simulink model "c00010M_harness"  (R2018a)
settings: Solver=FixedStepAuto  StartTime=0.0  StopTime=300  FixedStep=0.1  RelTol=1e-3
undefined symbols (not defined in the file): A1, hmax, PriorityTank, R1, R2, sigbuilder_block, TempThreshold
(part 5 of 40)

== system c00010M_harness/M143 ==
  note: VALUES
      | ---------------------------------
      | ControlType = 1 | 2 | 3
      | FillTank = 0 | 1
      | EmptyTank = 0 | 1
      | ManualReference between 0 and 1
      | Tempreature between 0 and 100
      | EmergencyButton = 0 | 1
      | LiquidLevel between 0 and 1 (hmax)
  note: Inputs For Tank2
  note: NAMES
      | --------------------------------------------
      | CT1 = ControlType Tank 1
      | F1 = Fill Tank 1
      | E1 = Empty Tank 1
      | MR1 = Manual Reference Tank1
      | T1 = Temperature Tank 1
      | EB1 = Emergency Button Tank 1
      | LL1 = Liquid Level 1
  note: Inputs For Tank3
  note: Inputs For Tank1
  CT2 : Inport
  F2 : Inport  Port=2
  E2 : Inport  Port=3
  T2 : Inport  Port=4
  EB2 : Inport  Port=5
  CT3 : Inport  Port=6
  F3 : Inport  Port=7
  E3 : Inport  Port=8
  MR3 : Inport  Port=9
  T3 : Inport  Port=10
  EB3 : Inport  Port=11
  Tank2 : Subsystem
  Tank3 : Subsystem
  LL2 : Outport
  LL3 : Outport  Port=2
  wires:
  Tank2/1(LL2) -> LL2/1, Tank3/7(LL2)
  Tank3/1(LL3) -> LL3/1, Tank2/6(LL3)
  EB2/1 -> Tank2/5(EB2)
  MR3/1 -> Tank3/4(MR3)
  CT2/1 -> Tank2/1(CT2)
  F2/1 -> Tank2/2(F2)
  E3/1 -> Tank3/3(E3)
  E2/1 -> Tank2/3(E2)
  T2/1 -> Tank2/4(T2)
  CT3/1 -> Tank3/1(CT3)
  F3/1 -> Tank3/2(F3)
  EB3/1 -> Tank3/6(EB3)
  T3/1 -> Tank3/5(T3)

== system c00010M_harness/M144 ==
  note: VALUES
      | ---------------------------------
      | ControlType = 1 | 2 | 3
      | FillTank = 0 | 1
      | EmptyTank = 0 | 1
      | ManualReference between 0 and 1
      | Tempreature between 0 and 100
      | EmergencyButton = 0 | 1
      | LiquidLevel between 0 and 1 (hmax)
  note: Inputs For Tank2
  note: NAMES
      | --------------------------------------------
      | CT1 = ControlType Tank 1
      | F1 = Fill Tank 1
      | E1 = Empty Tank 1
      | MR1 = Manual Reference Tank1
      | T1 = Temperature Tank 1
      | EB1 = Emergency Button Tank 1
      | LL1 = Liquid Level 1
  note: Inputs For Tank3
  note: Inputs For Tank1
  CT2 : Inport
  F2 : Inport  Port=2
  E2 : Inport  Port=3
  T2 : Inport  Port=4
  EB2 : Inport  Port=5
  CT3 : Inport  Port=6
  F3 : Inport  Port=7
  E3 : Inport  Port=8
  MR3 : Inport  Port=9
  T3 : Inport  Port=10
  EB3 : Inport  Port=11
  Tank2 : Subsystem
  Tank3 : Subsystem
  LL2 : Outport
  LL3 : Outport  Port=2
  wires:
  Tank2/1(LL2) -> LL2/1, Tank3/7(LL2)
  Tank3/1(LL3) -> LL3/1, Tank2/6(LL3)
  EB2/1 -> Tank2/5(EB2)
  MR3/1 -> Tank3/4(MR3)
  CT2/1 -> Tank2/1(CT2)
  F2/1 -> Tank2/2(F2)
  E3/1 -> Tank3/3(E3)
  E2/1 -> Tank2/3(E2)
  T2/1 -> Tank2/4(T2)
  CT3/1 -> Tank3/1(CT3)
  F3/1 -> Tank3/2(F3)
  EB3/1 -> Tank3/6(EB3)
  T3/1 -> Tank3/5(T3)

== system c00010M_harness/M145 ==
  note: VALUES
      | ---------------------------------
      | ControlType = 1 | 2 | 3
      | FillTank = 0 | 1
      | EmptyTank = 0 | 1
      | ManualReference between 0 and 1
      | Tempreature between 0 and 100
      | EmergencyButton = 0 | 1
      | LiquidLevel between 0 and 1 (hmax)
  note: Inputs For Tank2
  note: NAMES
      | --------------------------------------------
      | CT1 = ControlType Tank 1
      | F1 = Fill Tank 1
      | E1 = Empty Tank 1
      | MR1 = Manual Reference Tank1
      | T1 = Temperature Tank 1
      | EB1 = Emergency Button Tank 1
      | LL1 = Liquid Level 1
  note: Inputs For Tank3
  note: Inputs For Tank1
  CT2 : Inport
  F2 : Inport  Port=2
  E2 : Inport  Port=3
  T2 : Inport  Port=4
  EB2 : Inport  Port=5
  CT3 : Inport  Port=6
  F3 : Inport  Port=7
  E3 : Inport  Port=8
  MR3 : Inport  Port=9
  T3 : Inport  Port=10
  EB3 : Inport  Port=11
  Tank2 : Subsystem
  Tank3 : Subsystem
  LL2 : Outport
  LL3 : Outport  Port=2
  wires:
  Tank2/1(LL2) -> LL2/1, Tank3/7(LL2)
  Tank3/1(LL3) -> LL3/1, Tank2/6(LL3)
  EB2/1 -> Tank2/5(EB2)
  MR3/1 -> Tank3/4(MR3)
  CT2/1 -> Tank2/1(CT2)
  F2/1 -> Tank2/2(F2)
  E3/1 -> Tank3/3(E3)
  E2/1 -> Tank2/3(E2)
  T2/1 -> Tank2/4(T2)
  CT3/1 -> Tank3/1(CT3)
  F3/1 -> Tank3/2(F3)
  EB3/1 -> Tank3/6(EB3)
  T3/1 -> Tank3/5(T3)

== system c00010M_harness/M146 ==
  note: VALUES
      | ---------------------------------
      | ControlType = 1 | 2 | 3
      | FillTank = 0 | 1
      | EmptyTank = 0 | 1
      | ManualReference between 0 and 1
      | Tempreature between 0 and 100
      | EmergencyButton = 0 | 1
      | LiquidLevel between 0 and 1 (hmax)
  note: Inputs For Tank2
  note: NAMES
      | --------------------------------------------
      | CT1 = ControlType Tank 1
      | F1 = Fill Tank 1
      | E1 = Empty Tank 1
      | MR1 = Manual Reference Tank1
      | T1 = Temperature Tank 1
      | EB1 = Emergency Button Tank 1
      | LL1 = Liquid Level 1
  note: Inputs For Tank3
  note: Inputs For Tank1
  CT2 : Inport
  F2 : Inport  Port=2
  E2 : Inport  Port=3
  T2 : Inport  Port=4
  EB2 : Inport  Port=5
  CT3 : Inport  Port=6
  F3 : Inport  Port=7
  E3 : Inport  Port=8
  MR3 : Inport  Port=9
  T3 : Inport  Port=10
  EB3 : Inport  Port=11
  Tank2 : Subsystem
  Tank3 : Subsystem
  LL2 : Outport
  LL3 : Outport  Port=2
  wires:
  Tank2/1(LL2) -> LL2/1, Tank3/7(LL2)
  Tank3/1(LL3) -> LL3/1, Tank2/6(LL3)
  EB2/1 -> Tank2/5(EB2)
  MR3/1 -> Tank3/4(MR3)
  CT2/1 -> Tank2/1(CT2)
  F2/1 -> Tank2/2(F2)
  E3/1 -> Tank3/3(E3)
  E2/1 -> Tank2/3(E2)
  T2/1 -> Tank2/4(T2)
  CT3/1 -> Tank3/1(CT3)
  F3/1 -> Tank3/2(F3)
  EB3/1 -> Tank3/6(EB3)
  T3/1 -> Tank3/5(T3)

== system c00010M_harness/M147 ==
  note: VALUES
      | ---------------------------------
      | ControlType = 1 | 2 | 3
      | FillTank = 0 | 1
      | EmptyTank = 0 | 1
      | ManualReference between 0 and 1
      | Tempreature between 0 and 100
      | EmergencyButton = 0 | 1
      | LiquidLevel between 0 and 1 (hmax)
  note: Inputs For Tank2
  note: NAMES
      | --------------------------------------------
      | CT1 = ControlType Tank 1
      | F1 = Fill Tank 1
      | E1 = Empty Tank 1
      | MR1 = Manual Reference Tank1
      | T1 = Temperature Tank 1
      | EB1 = Emergency Button Tank 1
      | LL1 = Liquid Level 1
  note: Inputs For Tank3
  note: Inputs For Tank1
  CT2 : Inport
  F2 : Inport  Port=2
  E2 : Inport  Port=3
  T2 : Inport  Port=4
  EB2 : Inport  Port=5
  CT3 : Inport  Port=6
  F3 : Inport  Port=7
  E3 : Inport  Port=8
  MR3 : Inport  Port=9
  T3 : Inport  Port=10
  EB3 : Inport  Port=11
  Tank2 : Subsystem
  Tank3 : Subsystem
  LL2 : Outport
  LL3 : Outport  Port=2
  wires:
  Tank2/1(LL2) -> LL2/1, Tank3/7(LL2)
  Tank3/1(LL3) -> LL3/1, Tank2/6(LL3)
  EB2/1 -> Tank2/5(EB2)
  MR3/1 -> Tank3/4(MR3)
  CT2/1 -> Tank2/1(CT2)
  F2/1 -> Tank2/2(F2)
  E3/1 -> Tank3/3(E3)
  E2/1 -> Tank2/3(E2)
  T2/1 -> Tank2/4(T2)
  CT3/1 -> Tank3/1(CT3)
  F3/1 -> Tank3/2(F3)
  EB3/1 -> Tank3/6(EB3)
  T3/1 -> Tank3/5(T3)

== system c00010M_harness/M148 ==
  note: VALUES
      | ---------------------------------
      | ControlType = 1 | 2 | 3
      | FillTank = 0 | 1
      | EmptyTank = 0 | 1
      | ManualReference between 0 and 1
      | Tempreature between 0 and 100
      | EmergencyButton = 0 | 1
      | LiquidLevel between 0 and 1 (hmax)
  note: Inputs For Tank2
  note: NAMES
      | --------------------------------------------
      | CT1 = ControlType Tank 1
      | F1 = Fill Tank 1
      | E1 = Empty Tank 1
      | MR1 = Manual Reference Tank1
      | T1 = Temperature Tank 1
      | EB1 = Emergency Button Tank 1
      | LL1 = Liquid Level 1
  note: Inputs For Tank3
  note: Inputs For Tank1
  CT2 : Inport
  F2 : Inport  Port=2
  E2 : Inport  Port=3
  T2 : Inport  Port=4
  EB2 : Inport  Port=5
  CT3 : Inport  Port=6
  F3 : Inport  Port=7
  E3 : Inport  Port=8
  MR3 : Inport  Port=9
  T3 : Inport  Port=10
  EB3 : Inport  Port=11
  Tank2 : Subsystem
  Tank3 : Subsystem
  LL2 : Outport
  LL3 : Outport  Port=2
  wires:
  Tank2/1(LL2) -> LL2/1, Tank3/7(LL2)
  Tank3/1(LL3) -> LL3/1, Tank2/6(LL3)
  EB2/1 -> Tank2/5(EB2)
  MR3/1 -> Tank3/4(MR3)
  CT2/1 -> Tank2/1(CT2)
  F2/1 -> Tank2/2(F2)
  E3/1 -> Tank3/3(E3)
  E2/1 -> Tank2/3(E2)
  T2/1 -> Tank2/4(T2)
  CT3/1 -> Tank3/1(CT3)
  F3/1 -> Tank3/2(F3)
  EB3/1 -> Tank3/6(EB3)
  T3/1 -> Tank3/5(T3)

== system c00010M_harness/M149 ==
  note: VALUES
      | ---------------------------------
      | ControlType = 1 | 2 | 3
      | FillTank = 0 | 1
      | EmptyTank = 0 | 1
      | ManualReference between 0 and 1
      | Tempreature between 0 and 100
      | EmergencyButton = 0 | 1
      | LiquidLevel between 0 and 1 (hmax)
  note: Inputs For Tank2
  note: NAMES
      | --------------------------------------------
      | CT1 = ControlType Tank 1
      | F1 = Fill Tank 1
      | E1 = Empty Tank 1
      | MR1 = Manual Reference Tank1
      | T1 = Temperature Tank 1
      | EB1 = Emergency Button Tank 1
      | LL1 = Liquid Level 1
  note: Inputs For Tank3
  note: Inputs For Tank1
  CT2 : Inport
  F2 : Inport  Port=2
  E2 : Inport  Port=3
  T2 : Inport  Port=4
  EB2 : Inport  Port=5
  CT3 : Inport  Port=6
  F3 : Inport  Port=7
  E3 : Inport  Port=8
  MR3 : Inport  Port=9
  T3 : Inport  Port=10
  EB3 : Inport  Port=11
  Tank2 : Subsystem
  Tank3 : Subsystem
  LL2 : Outport
  LL3 : Outport  Port=2
  wires:
  Tank2/1(LL2) -> LL2/1, Tank3/7(LL2)
  Tank3/1(LL3) -> LL3/1, Tank2/6(LL3)
  EB2/1 -> Tank2/5(EB2)
  MR3/1 -> Tank3/4(MR3)
  CT2/1 -> Tank2/1(CT2)
  F2/1 -> Tank2/2(F2)
  E3/1 -> Tank3/3(E3)
  E2/1 -> Tank2/3(E2)
  T2/1 -> Tank2/4(T2)
  CT3/1 -> Tank3/1(CT3)
  F3/1 -> Tank3/2(F3)
  EB3/1 -> Tank3/6(EB3)
  T3/1 -> Tank3/5(T3)

== system c00010M_harness/M150 ==
  note: VALUES
      | ---------------------------------
      | ControlType = 1 | 2 | 3
      | FillTank = 0 | 1
      | EmptyTank = 0 | 1
      | ManualReference between 0 and 1
      | Tempreature between 0 and 100
      | EmergencyButton = 0 | 1
      | LiquidLevel between 0 and 1 (hmax)
  note: Inputs For Tank2
  note: NAMES
      | --------------------------------------------
      | CT1 = ControlType Tank 1
      | F1 = Fill Tank 1
      | E1 = Empty Tank 1
      | MR1 = Manual Reference Tank1
      | T1 = Temperature Tank 1
      | EB1 = Emergency Button Tank 1
      | LL1 = Liquid Level 1
  note: Inputs For Tank3
  note: Inputs For Tank1
  CT2 : Inport
  F2 : Inport  Port=2
  E2 : Inport  Port=3
  T2 : Inport  Port=4
  EB2 : Inport  Port=5
  CT3 : Inport  Port=6
  F3 : Inport  Port=7
  E3 : Inport  Port=8
  MR3 : Inport  Port=9
  T3 : Inport  Port=10
  EB3 : Inport  Port=11
  Tank2 : Subsystem
  Tank3 : Subsystem
  LL2 : Outport
  LL3 : Outport  Port=2
  wires:
  Tank2/1(LL2) -> LL2/1, Tank3/7(LL2)
  Tank3/1(LL3) -> LL3/1, Tank2/6(LL3)
  EB2/1 -> Tank2/5(EB2)
  MR3/1 -> Tank3/4(MR3)
  CT2/1 -> Tank2/1(CT2)
  F2/1 -> Tank2/2(F2)
  E3/1 -> Tank3/3(E3)
  E2/1 -> Tank2/3(E2)
  T2/1 -> Tank2/4(T2)
  CT3/1 -> Tank3/1(CT3)
  F3/1 -> Tank3/2(F3)
  EB3/1 -> Tank3/6(EB3)
  T3/1 -> Tank3/5(T3)

== system c00010M_harness/M151 ==
  note: VALUES
      | ---------------------------------
      | ControlType = 1 | 2 | 3
      | FillTank = 0 | 1
      | EmptyTank = 0 | 1
      | ManualReference between 0 and 1
      | Tempreature between 0 and 100
      | EmergencyButton = 0 | 1
      | LiquidLevel between 0 and 1 (hmax)
  note: Inputs For Tank2
  note: NAMES
      | --------------------------------------------
      | CT1 = ControlType Tank 1
      | F1 = Fill Tank 1
      | E1 = Empty Tank 1
      | MR1 = Manual Reference Tank1
      | T1 = Temperature Tank 1
      | EB1 = Emergency Button Tank 1
      | LL1 = Liquid Level 1
  note: Inputs For Tank3
  note: Inputs For Tank1
  CT2 : Inport
  F2 : Inport  Port=2
  E2 : Inport  Port=3
  T2 : Inport  Port=4
  EB2 : Inport  Port=5
  CT3 : Inport  Port=6
  F3 : Inport  Port=7
  E3 : Inport  Port=8
  MR3 : Inport  Port=9
  T3 : Inport  Port=10
  EB3 : Inport  Port=11
  Tank2 : Subsystem
  Tank3 : Subsystem
  LL2 : Outport
  LL3 : Outport  Port=2
  wires:
  Tank2/1(LL2) -> LL2/1, Tank3/7(LL2)
  Tank3/1(LL3) -> LL3/1, Tank2/6(LL3)
  EB2/1 -> Tank2/5(EB2)
  MR3/1 -> Tank3/4(MR3)
  CT2/1 -> Tank2/1(CT2)
  F2/1 -> Tank2/2(F2)
  E3/1 -> Tank3/3(E3)
  E2/1 -> Tank2/3(E2)
  T2/1 -> Tank2/4(T2)
  CT3/1 -> Tank3/1(CT3)
  F3/1 -> Tank3/2(F3)
  EB3/1 -> Tank3/6(EB3)
  T3/1 -> Tank3/5(T3)

== system c00010M_harness/M152 ==
  note: VALUES
      | ---------------------------------
      | ControlType = 1 | 2 | 3
      | FillTank = 0 | 1
      | EmptyTank = 0 | 1
      | ManualReference between 0 and 1
      | Tempreature between 0 and 100
      | EmergencyButton = 0 | 1
      | LiquidLevel between 0 and 1 (hmax)
  note: Inputs For Tank2
  note: NAMES
      | --------------------------------------------
      | CT1 = ControlType Tank 1
      | F1 = Fill Tank 1
      | E1 = Empty Tank 1
      | MR1 = Manual Reference Tank1
      | T1 = Temperature Tank 1
      | EB1 = Emergency Button Tank 1
      | LL1 = Liquid Level 1
  note: Inputs For Tank3
  note: Inputs For Tank1
  CT2 : Inport
  F2 : Inport  Port=2
  E2 : Inport  Port=3
  T2 : Inport  Port=4
  EB2 : Inport  Port=5
  CT3 : Inport  Port=6
  F3 : Inport  Port=7
  E3 : Inport  Port=8
  MR3 : Inport  Port=9
  T3 : Inport  Port=10
  EB3 : Inport  Port=11
  Tank2 : Subsystem
  Tank3 : Subsystem
  LL2 : Outport
  LL3 : Outport  Port=2
  wires:
  Tank2/1(LL2) -> LL2/1, Tank3/7(LL2)
  Tank3/1(LL3) -> LL3/1, Tank2/6(LL3)
  EB2/1 -> Tank2/5(EB2)
  MR3/1 -> Tank3/4(MR3)
  CT2/1 -> Tank2/1(CT2)
  F2/1 -> Tank2/2(F2)
  E3/1 -> Tank3/3(E3)
  E2/1 -> Tank2/3(E2)
  T2/1 -> Tank2/4(T2)
  CT3/1 -> Tank3/1(CT3)
  F3/1 -> Tank3/2(F3)
  EB3/1 -> Tank3/6(EB3)
  T3/1 -> Tank3/5(T3)

== system c00010M_harness/M153 ==
  note: VALUES
      | ---------------------------------
      | ControlType = 1 | 2 | 3
      | FillTank = 0 | 1
      | EmptyTank = 0 | 1
      | ManualReference between 0 and 1
      | Tempreature between 0 and 100
      | EmergencyButton = 0 | 1
      | LiquidLevel between 0 and 1 (hmax)
  note: Inputs For Tank2
  note: NAMES
      | --------------------------------------------
      | CT1 = ControlType Tank 1
      | F1 = Fill Tank 1
      | E1 = Empty Tank 1
      | MR1 = Manual Reference Tank1
      | T1 = Temperature Tank 1
      | EB1 = Emergency Button Tank 1
      | LL1 = Liquid Level 1
  note: Inputs For Tank3
  note: Inputs For Tank1
  CT2 : Inport
  F2 : Inport  Port=2
  E2 : Inport  Port=3
  T2 : Inport  Port=4
  EB2 : Inport  Port=5
  CT3 : Inport  Port=6
  F3 : Inport  Port=7
  E3 : Inport  Port=8
  MR3 : Inport  Port=9
  T3 : Inport  Port=10
  EB3 : Inport  Port=11
  Tank2 : Subsystem
  Tank3 : Subsystem
  LL2 : Outport
  LL3 : Outport  Port=2
  wires:
  Tank2/1(LL2) -> LL2/1, Tank3/7(LL2)
  Tank3/1(LL3) -> LL3/1, Tank2/6(LL3)
  EB2/1 -> Tank2/5(EB2)
  MR3/1 -> Tank3/4(MR3)
  CT2/1 -> Tank2/1(CT2)
  F2/1 -> Tank2/2(F2)
  E3/1 -> Tank3/3(E3)
  E2/1 -> Tank2/3(E2)
  T2/1 -> Tank2/4(T2)
  CT3/1 -> Tank3/1(CT3)
  F3/1 -> Tank3/2(F3)
  EB3/1 -> Tank3/6(EB3)
  T3/1 -> Tank3/5(T3)

== system c00010M_harness/M154 ==
  note: VALUES
      | ---------------------------------
      | ControlType = 1 | 2 | 3
      | FillTank = 0 | 1
      | EmptyTank = 0 | 1
      | ManualReference between 0 and 1
      | Tempreature between 0 and 100
      | EmergencyButton = 0 | 1
      | LiquidLevel between 0 and 1 (hmax)
  note: Inputs For Tank2
  note: NAMES
      | --------------------------------------------
      | CT1 = ControlType Tank 1
      | F1 = Fill Tank 1
      | E1 = Empty Tank 1
      | MR1 = Manual Reference Tank1
      | T1 = Temperature Tank 1
      | EB1 = Emergency Button Tank 1
      | LL1 = Liquid Level 1
  note: Inputs For Tank3
  note: Inputs For Tank1
  CT2 : Inport
  F2 : Inport  Port=2
  E2 : Inport  Port=3
  T2 : Inport  Port=4
  EB2 : Inport  Port=5
  CT3 : Inport  Port=6
  F3 : Inport  Port=7
  E3 : Inport  Port=8
  MR3 : Inport  Port=9
  T3 : Inport  Port=10
  EB3 : Inport  Port=11
  Tank2 : Subsystem
  Tank3 : Subsystem
  LL2 : Outport
  LL3 : Outport  Port=2
  wires:
  Tank2/1(LL2) -> LL2/1, Tank3/7(LL2)
  Tank3/1(LL3) -> LL3/1, Tank2/6(LL3)
  EB2/1 -> Tank2/5(EB2)
  MR3/1 -> Tank3/4(MR3)
  CT2/1 -> Tank2/1(CT2)
  F2/1 -> Tank2/2(F2)
  E3/1 -> Tank3/3(E3)
  E2/1 -> Tank2/3(E2)
  T2/1 -> Tank2/4(T2)
  CT3/1 -> Tank3/1(CT3)
  F3/1 -> Tank3/2(F3)
  EB3/1 -> Tank3/6(EB3)
  T3/1 -> Tank3/5(T3)

== system c00010M_harness/M155 ==
  note: VALUES
      | ---------------------------------
      | ControlType = 1 | 2 | 3
      | FillTank = 0 | 1
      | EmptyTank = 0 | 1
      | ManualReference between 0 and 1
      | Tempreature between 0 and 100
      | EmergencyButton = 0 | 1
      | LiquidLevel between 0 and 1 (hmax)
  note: Inputs For Tank2
  note: NAMES
      | --------------------------------------------
      | CT1 = ControlType Tank 1
      | F1 = Fill Tank 1
      | E1 = Empty Tank 1
      | MR1 = Manual Reference Tank1
      | T1 = Temperature Tank 1
      | EB1 = Emergency Button Tank 1
      | LL1 = Liquid Level 1
  note: Inputs For Tank3
  note: Inputs For Tank1
  CT2 : Inport
  F2 : Inport  Port=2
  E2 : Inport  Port=3
  T2 : Inport  Port=4
  EB2 : Inport  Port=5
  CT3 : Inport  Port=6
  F3 : Inport  Port=7
  E3 : Inport  Port=8
  MR3 : Inport  Port=9
  T3 : Inport  Port=10
  EB3 : Inport  Port=11
  Tank2 : Subsystem
  Tank3 : Subsystem
  LL2 : Outport
  LL3 : Outport  Port=2
  wires:
  Tank2/1(LL2) -> LL2/1, Tank3/7(LL2)
  Tank3/1(LL3) -> LL3/1, Tank2/6(LL3)
  EB2/1 -> Tank2/5(EB2)
  MR3/1 -> Tank3/4(MR3)
  CT2/1 -> Tank2/1(CT2)
  F2/1 -> Tank2/2(F2)
  E3/1 -> Tank3/3(E3)
  E2/1 -> Tank2/3(E2)
  T2/1 -> Tank2/4(T2)
  CT3/1 -> Tank3/1(CT3)
  F3/1 -> Tank3/2(F3)
  EB3/1 -> Tank3/6(EB3)
  T3/1 -> Tank3/5(T3)

== system c00010M_harness/M156 ==
  note: VALUES
      | ---------------------------------
      | ControlType = 1 | 2 | 3
      | FillTank = 0 | 1
      | EmptyTank = 0 | 1
      | ManualReference between 0 and 1
      | Tempreature between 0 and 100
      | EmergencyButton = 0 | 1
      | LiquidLevel between 0 and 1 (hmax)
  note: Inputs For Tank2
  note: NAMES
      | --------------------------------------------
      | CT1 = ControlType Tank 1
      | F1 = Fill Tank 1
      | E1 = Empty Tank 1
      | MR1 = Manual Reference Tank1
      | T1 = Temperature Tank 1
      | EB1 = Emergency Button Tank 1
      | LL1 = Liquid Level 1
  note: Inputs For Tank3
  note: Inputs For Tank1
  CT2 : Inport
  F2 : Inport  Port=2
  E2 : Inport  Port=3
  T2 : Inport  Port=4
  EB2 : Inport  Port=5
  CT3 : Inport  Port=6
  F3 : Inport  Port=7
  E3 : Inport  Port=8
  MR3 : Inport  Port=9
  T3 : Inport  Port=10
  EB3 : Inport  Port=11
  Tank2 : Subsystem
  Tank3 : Subsystem
  LL2 : Outport
  LL3 : Outport  Port=2
  wires:
  Tank2/1(LL2) -> LL2/1, Tank3/7(LL2)
  Tank3/1(LL3) -> LL3/1, Tank2/6(LL3)
  EB2/1 -> Tank2/5(EB2)
  MR3/1 -> Tank3/4(MR3)
  CT2/1 -> Tank2/1(CT2)
  F2/1 -> Tank2/2(F2)
  E3/1 -> Tank3/3(E3)
  E2/1 -> Tank2/3(E2)
  T2/1 -> Tank2/4(T2)
  CT3/1 -> Tank3/1(CT3)
  F3/1 -> Tank3/2(F3)
  EB3/1 -> Tank3/6(EB3)
  T3/1 -> Tank3/5(T3)

== system c00010M_harness/M157 ==
  note: VALUES
      | ---------------------------------
      | ControlType = 1 | 2 | 3
      | FillTank = 0 | 1
      | EmptyTank = 0 | 1
      | ManualReference between 0 and 1
      | Tempreature between 0 and 100
      | EmergencyButton = 0 | 1
      | LiquidLevel between 0 and 1 (hmax)
  note: Inputs For Tank2
  note: NAMES
      | --------------------------------------------
      | CT1 = ControlType Tank 1
      | F1 = Fill Tank 1
      | E1 = Empty Tank 1
      | MR1 = Manual Reference Tank1
      | T1 = Temperature Tank 1
      | EB1 = Emergency Button Tank 1
      | LL1 = Liquid Level 1
  note: Inputs For Tank3
  note: Inputs For Tank1
  CT2 : Inport
  F2 : Inport  Port=2
  E2 : Inport  Port=3
  T2 : Inport  Port=4
  EB2 : Inport  Port=5
  CT3 : Inport  Port=6
  F3 : Inport  Port=7
  E3 : Inport  Port=8
  MR3 : Inport  Port=9
  T3 : Inport  Port=10
  EB3 : Inport  Port=11
  Tank2 : Subsystem
  Tank3 : Subsystem
  LL2 : Outport
  LL3 : Outport  Port=2
  wires:
  Tank2/1(LL2) -> LL2/1, Tank3/7(LL2)
  Tank3/1(LL3) -> LL3/1, Tank2/6(LL3)
  EB2/1 -> Tank2/5(EB2)
  MR3/1 -> Tank3/4(MR3)
  CT2/1 -> Tank2/1(CT2)
  F2/1 -> Tank2/2(F2)
  E3/1 -> Tank3/3(E3)
  E2/1 -> Tank2/3(E2)
  T2/1 -> Tank2/4(T2)
  CT3/1 -> Tank3/1(CT3)
  F3/1 -> Tank3/2(F3)
  EB3/1 -> Tank3/6(EB3)
  T3/1 -> Tank3/5(T3)

== system c00010M_harness/M158 ==
  note: VALUES
      | ---------------------------------
      | ControlType = 1 | 2 | 3
      | FillTank = 0 | 1
      | EmptyTank = 0 | 1
      | ManualReference between 0 and 1
      | Tempreature between 0 and 100
      | EmergencyButton = 0 | 1
      | LiquidLevel between 0 and 1 (hmax)
  note: Inputs For Tank2
  note: NAMES
      | --------------------------------------------
      | CT1 = ControlType Tank 1
      | F1 = Fill Tank 1
      | E1 = Empty Tank 1
      | MR1 = Manual Reference Tank1
      | T1 = Temperature Tank 1
      | EB1 = Emergency Button Tank 1
      | LL1 = Liquid Level 1
  note: Inputs For Tank3
  note: Inputs For Tank1
  CT2 : Inport
  F2 : Inport  Port=2
  E2 : Inport  Port=3
  T2 : Inport  Port=4
  EB2 : Inport  Port=5
  CT3 : Inport  Port=6
  F3 : Inport  Port=7
  E3 : Inport  Port=8
  MR3 : Inport  Port=9
  T3 : Inport  Port=10
  EB3 : Inport  Port=11
  Tank2 : Subsystem
  Tank3 : Subsystem
  LL2 : Outport
  LL3 : Outport  Port=2
  wires:
  Tank2/1(LL2) -> LL2/1, Tank3/7(LL2)
  Tank3/1(LL3) -> LL3/1, Tank2/6(LL3)
  EB2/1 -> Tank2/5(EB2)
  MR3/1 -> Tank3/4(MR3)
  CT2/1 -> Tank2/1(CT2)
  F2/1 -> Tank2/2(F2)
  E3/1 -> Tank3/3(E3)
  E2/1 -> Tank2/3(E2)
  T2/1 -> Tank2/4(T2)
  CT3/1 -> Tank3/1(CT3)
  F3/1 -> Tank3/2(F3)
  EB3/1 -> Tank3/6(EB3)
  T3/1 -> Tank3/5(T3)

== system c00010M_harness/M159 ==
  note: VALUES
      | ---------------------------------
      | ControlType = 1 | 2 | 3
      | FillTank = 0 | 1
      | EmptyTank = 0 | 1
      | ManualReference between 0 and 1
      | Tempreature between 0 and 100
      | EmergencyButton = 0 | 1
      | LiquidLevel between 0 and 1 (hmax)
  note: Inputs For Tank2
  note: NAMES
      | --------------------------------------------
      | CT1 = ControlType Tank 1
      | F1 = Fill Tank 1
      | E1 = Empty Tank 1
      | MR1 = Manual Reference Tank1
      | T1 = Temperature Tank 1
      | EB1 = Emergency Button Tank 1
      | LL1 = Liquid Level 1
  note: Inputs For Tank3
  note: Inputs For Tank1
  CT2 : Inport
  F2 : Inport  Port=2
  E2 : Inport  Port=3
  T2 : Inport  Port=4
  EB2 : Inport  Port=5
  CT3 : Inport  Port=6
  F3 : Inport  Port=7
  E3 : Inport  Port=8
  MR3 : Inport  Port=9
  T3 : Inport  Port=10
  EB3 : Inport  Port=11
  Tank2 : Subsystem
  Tank3 : Subsystem
  LL2 : Outport
  LL3 : Outport  Port=2
  wires:
  Tank2/1(LL2) -> LL2/1, Tank3/7(LL2)
  Tank3/1(LL3) -> LL3/1, Tank2/6(LL3)
  EB2/1 -> Tank2/5(EB2)
  MR3/1 -> Tank3/4(MR3)
  CT2/1 -> Tank2/1(CT2)
  F2/1 -> Tank2/2(F2)
  E3/1 -> Tank3/3(E3)
  E2/1 -> Tank2/3(E2)
  T2/1 -> Tank2/4(T2)
  CT3/1 -> Tank3/1(CT3)
  F3/1 -> Tank3/2(F3)
  EB3/1 -> Tank3/6(EB3)
  T3/1 -> Tank3/5(T3)

== system c00010M_harness/M160 ==
  note: VALUES
      | ---------------------------------
      | ControlType = 1 | 2 | 3
      | FillTank = 0 | 1
      | EmptyTank = 0 | 1
      | ManualReference between 0 and 1
      | Tempreature between 0 and 100
      | EmergencyButton = 0 | 1
      | LiquidLevel between 0 and 1 (hmax)
  note: Inputs For Tank2
  note: NAMES
      | --------------------------------------------
      | CT1 = ControlType Tank 1
      | F1 = Fill Tank 1
      | E1 = Empty Tank 1
      | MR1 = Manual Reference Tank1
      | T1 = Temperature Tank 1
      | EB1 = Emergency Button Tank 1
      | LL1 = Liquid Level 1
  note: Inputs For Tank3
  note: Inputs For Tank1
  CT2 : Inport
  F2 : Inport  Port=2
  E2 : Inport  Port=3
  T2 : Inport  Port=4
  EB2 : Inport  Port=5
  CT3 : Inport  Port=6
  F3 : Inport  Port=7
  E3 : Inport  Port=8
  MR3 : Inport  Port=9
  T3 : Inport  Port=10
  EB3 : Inport  Port=11
  Tank2 : Subsystem
  Tank3 : Subsystem
  LL2 : Outport
  LL3 : Outport  Port=2
  wires:
  Tank2/1(LL2) -> LL2/1, Tank3/7(LL2)
  Tank3/1(LL3) -> LL3/1, Tank2/6(LL3)
  EB2/1 -> Tank2/5(EB2)
  MR3/1 -> Tank3/4(MR3)
  CT2/1 -> Tank2/1(CT2)
  F2/1 -> Tank2/2(F2)
  E3/1 -> Tank3/3(E3)
  E2/1 -> Tank2/3(E2)
  T2/1 -> Tank2/4(T2)
  CT3/1 -> Tank3/1(CT3)
  F3/1 -> Tank3/2(F3)
  EB3/1 -> Tank3/6(EB3)
  T3/1 -> Tank3/5(T3)

== system c00010M_harness/M161 ==
  note: VALUES
      | ---------------------------------
      | ControlType = 1 | 2 | 3
      | FillTank = 0 | 1
      | EmptyTank = 0 | 1
      | ManualReference between 0 and 1
      | Tempreature between 0 and 100
      | EmergencyButton = 0 | 1
      | LiquidLevel between 0 and 1 (hmax)
  note: Inputs For Tank2
  note: NAMES
      | --------------------------------------------
      | CT1 = ControlType Tank 1
      | F1 = Fill Tank 1
      | E1 = Empty Tank 1
      | MR1 = Manual Reference Tank1
      | T1 = Temperature Tank 1
      | EB1 = Emergency Button Tank 1
      | LL1 = Liquid Level 1
  note: Inputs For Tank3
  note: Inputs For Tank1
  CT2 : Inport
  F2 : Inport  Port=2
  E2 : Inport  Port=3
  T2 : Inport  Port=4
  EB2 : Inport  Port=5
  CT3 : Inport  Port=6
  F3 : Inport  Port=7
  E3 : Inport  Port=8
  MR3 : Inport  Port=9
  T3 : Inport  Port=10
  EB3 : Inport  Port=11
  Tank2 : Subsystem
  Tank3 : Subsystem
  LL2 : Outport
  LL3 : Outport  Port=2
  wires:
  Tank2/1(LL2) -> LL2/1, Tank3/7(LL2)
  Tank3/1(LL3) -> LL3/1, Tank2/6(LL3)
  EB2/1 -> Tank2/5(EB2)
  MR3/1 -> Tank3/4(MR3)
  CT2/1 -> Tank2/1(CT2)
  F2/1 -> Tank2/2(F2)
  E3/1 -> Tank3/3(E3)
  E2/1 -> Tank2/3(E2)
  T2/1 -> Tank2/4(T2)
  CT3/1 -> Tank3/1(CT3)
  F3/1 -> Tank3/2(F3)
  EB3/1 -> Tank3/6(EB3)
  T3/1 -> Tank3/5(T3)

== system c00010M_harness/M162 ==
  note: VALUES
      | ---------------------------------
      | ControlType = 1 | 2 | 3
      | FillTank = 0 | 1
      | EmptyTank = 0 | 1
      | ManualReference between 0 and 1
      | Tempreature between 0 and 100
      | EmergencyButton = 0 | 1
      | LiquidLevel between 0 and 1 (hmax)
  note: Inputs For Tank2
  note: NAMES
      | --------------------------------------------
      | CT1 = ControlType Tank 1
      | F1 = Fill Tank 1
      | E1 = Empty Tank 1
      | MR1 = Manual Reference Tank1
      | T1 = Temperature Tank 1
      | EB1 = Emergency Button Tank 1
      | LL1 = Liquid Level 1
  note: Inputs For Tank3
  note: Inputs For Tank1
  CT2 : Inport
  F2 : Inport  Port=2
  E2 : Inport  Port=3
  T2 : Inport  Port=4
  EB2 : Inport  Port=5
  CT3 : Inport  Port=6
  F3 : Inport  Port=7
  E3 : Inport  Port=8
  MR3 : Inport  Port=9
  T3 : Inport  Port=10
  EB3 : Inport  Port=11
  Tank2 : Subsystem
  Tank3 : Subsystem
  LL2 : Outport
  LL3 : Outport  Port=2
  wires:
  Tank2/1(LL2) -> LL2/1, Tank3/7(LL2)
  Tank3/1(LL3) -> LL3/1, Tank2/6(LL3)
  EB2/1 -> Tank2/5(EB2)
  MR3/1 -> Tank3/4(MR3)
  CT2/1 -> Tank2/1(CT2)
  F2/1 -> Tank2/2(F2)
  E3/1 -> Tank3/3(E3)
  E2/1 -> Tank2/3(E2)
  T2/1 -> Tank2/4(T2)
  CT3/1 -> Tank3/1(CT3)
  F3/1 -> Tank3/2(F3)
  EB3/1 -> Tank3/6(EB3)
  T3/1 -> Tank3/5(T3)

== system c00010M_harness/M163 ==
  note: VALUES
      | ---------------------------------
      | ControlType = 1 | 2 | 3
      | FillTank = 0 | 1
      | EmptyTank = 0 | 1
      | ManualReference between 0 and 1
      | Tempreature between 0 and 100
      | EmergencyButton = 0 | 1
      | LiquidLevel between 0 and 1 (hmax)
  note: Inputs For Tank2
  note: NAMES
      | --------------------------------------------
      | CT1 = ControlType Tank 1
      | F1 = Fill Tank 1
      | E1 = Empty Tank 1
      | MR1 = Manual Reference Tank1
      | T1 = Temperature Tank 1
      | EB1 = Emergency Button Tank 1
      | LL1 = Liquid Level 1
  note: Inputs For Tank3
  note: Inputs For Tank1
  CT2 : Inport
  F2 : Inport  Port=2
  E2 : Inport  Port=3
  T2 : Inport  Port=4
  EB2 : Inport  Port=5
  CT3 : Inport  Port=6
  F3 : Inport  Port=7
  E3 : Inport  Port=8
  MR3 : Inport  Port=9
  T3 : Inport  Port=10
  EB3 : Inport  Port=11
  Tank2 : Subsystem
  Tank3 : Subsystem
  LL2 : Outport
  LL3 : Outport  Port=2
  wires:
  Tank2/1(LL2) -> LL2/1, Tank3/7(LL2)
  Tank3/1(LL3) -> LL3/1, Tank2/6(LL3)
  EB2/1 -> Tank2/5(EB2)
  MR3/1 -> Tank3/4(MR3)
  CT2/1 -> Tank2/1(CT2)
  F2/1 -> Tank2/2(F2)
  E3/1 -> Tank3/3(E3)
  E2/1 -> Tank2/3(E2)
  T2/1 -> Tank2/4(T2)
  CT3/1 -> Tank3/1(CT3)
  F3/1 -> Tank3/2(F3)
  EB3/1 -> Tank3/6(EB3)
  T3/1 -> Tank3/5(T3)

== system c00010M_harness/M164 ==
  note: VALUES
      | ---------------------------------
      | ControlType = 1 | 2 | 3
      | FillTank = 0 | 1
      | EmptyTank = 0 | 1
      | ManualReference between 0 and 1
      | Tempreature between 0 and 100
      | EmergencyButton = 0 | 1
      | LiquidLevel between 0 and 1 (hmax)
  note: Inputs For Tank2
  note: NAMES
      | --------------------------------------------
      | CT1 = ControlType Tank 1
      | F1 = Fill Tank 1
      | E1 = Empty Tank 1
      | MR1 = Manual Reference Tank1
      | T1 = Temperature Tank 1
      | EB1 = Emergency Button Tank 1
      | LL1 = Liquid Level 1
  note: Inputs For Tank3
  note: Inputs For Tank1
  CT2 : Inport
  F2 : Inport  Port=2
  E2 : Inport  Port=3
  T2 : Inport  Port=4
  EB2 : Inport  Port=5
  CT3 : Inport  Port=6
  F3 : Inport  Port=7
  E3 : Inport  Port=8
  MR3 : Inport  Port=9
  T3 : Inport  Port=10
  EB3 : Inport  Port=11
  Tank2 : Subsystem
  Tank3 : Subsystem
  LL2 : Outport
  LL3 : Outport  Port=2
  wires:
  Tank2/1(LL2) -> LL2/1, Tank3/7(LL2)
  Tank3/1(LL3) -> LL3/1, Tank2/6(LL3)
  EB2/1 -> Tank2/5(EB2)
  MR3/1 -> Tank3/4(MR3)
  CT2/1 -> Tank2/1(CT2)
  F2/1 -> Tank2/2(F2)
  E3/1 -> Tank3/3(E3)
  E2/1 -> Tank2/3(E2)
  T2/1 -> Tank2/4(T2)
  CT3/1 -> Tank3/1(CT3)
  F3/1 -> Tank3/2(F3)
  EB3/1 -> Tank3/6(EB3)
  T3/1 -> Tank3/5(T3)

== system c00010M_harness/M165 ==
  note: VALUES
      | ---------------------------------
      | ControlType = 1 | 2 | 3
      | FillTank = 0 | 1
      | EmptyTank = 0 | 1
      | ManualReference between 0 and 1
      | Tempreature between 0 and 100
      | EmergencyButton = 0 | 1
      | LiquidLevel between 0 and 1 (hmax)
  note: Inputs For Tank2
  note: NAMES
      | --------------------------------------------
      | CT1 = ControlType Tank 1
      | F1 = Fill Tank 1
      | E1 = Empty Tank 1
      | MR1 = Manual Reference Tank1
      | T1 = Temperature Tank 1
      | EB1 = Emergency Button Tank 1
      | LL1 = Liquid Level 1
  note: Inputs For Tank3
  note: Inputs For Tank1
  CT2 : Inport
  F2 : Inport  Port=2
  E2 : Inport  Port=3
  T2 : Inport  Port=4
  EB2 : Inport  Port=5
  CT3 : Inport  Port=6
  F3 : Inport  Port=7
  E3 : Inport  Port=8
  MR3 : Inport  Port=9
  T3 : Inport  Port=10
  EB3 : Inport  Port=11
  Tank2 : Subsystem
  Tank3 : Subsystem
  LL2 : Outport
  LL3 : Outport  Port=2
  wires:
  Tank2/1(LL2) -> LL2/1, Tank3/7(LL2)
  Tank3/1(LL3) -> LL3/1, Tank2/6(LL3)
  EB2/1 -> Tank2/5(EB2)
  MR3/1 -> Tank3/4(MR3)
  CT2/1 -> Tank2/1(CT2)
  F2/1 -> Tank2/2(F2)
  E3/1 -> Tank3/3(E3)
  E2/1 -> Tank2/3(E2)
  T2/1 -> Tank2/4(T2)
  CT3/1 -> Tank3/1(CT3)
  F3/1 -> Tank3/2(F3)
  EB3/1 -> Tank3/6(EB3)
  T3/1 -> Tank3/5(T3)

== system c00010M_harness/M169 ==
  note: VALUES
      | ---------------------------------
      | ControlType = 1 | 2 | 3
      | FillTank = 0 | 1
      | EmptyTank = 0 | 1
      | ManualReference between 0 and 1
      | Tempreature between 0 and 100
      | EmergencyButton = 0 | 1
      | LiquidLevel between 0 and 1 (hmax)
  note: Inputs For Tank2
  note: NAMES
      | --------------------------------------------
      | CT1 = ControlType Tank 1
      | F1 = Fill Tank 1
      | E1 = Empty Tank 1
      | MR1 = Manual Reference Tank1
      | T1 = Temperature Tank 1
      | EB1 = Emergency Button Tank 1
      | LL1 = Liquid Level 1
  note: Inputs For Tank3
  note: Inputs For Tank1
  CT2 : Inport
  F2 : Inport  Port=2
  E2 : Inport  Port=3
  T2 : Inport  Port=4
  EB2 : Inport  Port=5
  CT3 : Inport  Port=6
  F3 : Inport  Port=7
  E3 : Inport  Port=8
  MR3 : Inport  Port=9
  T3 : Inport  Port=10
  EB3 : Inport  Port=11
  Tank2 : Subsystem
  Tank3 : Subsystem
  LL2 : Outport
  LL3 : Outport  Port=2
  wires:
  Tank2/1(LL2) -> LL2/1, Tank3/7(LL2)
  Tank3/1(LL3) -> LL3/1, Tank2/6(LL3)
  EB2/1 -> Tank2/5(EB2)
  MR3/1 -> Tank3/4(MR3)
  CT2/1 -> Tank2/1(CT2)
  F2/1 -> Tank2/2(F2)
  E3/1 -> Tank3/3(E3)
  E2/1 -> Tank2/3(E2)
  T2/1 -> Tank2/4(T2)
  CT3/1 -> Tank3/1(CT3)
  F3/1 -> Tank3/2(F3)
  EB3/1 -> Tank3/6(EB3)
  T3/1 -> Tank3/5(T3)

== system c00010M_harness/M170 ==
  note: VALUES
      | ---------------------------------
      | ControlType = 1 | 2 | 3
      | FillTank = 0 | 1
      | EmptyTank = 0 | 1
      | ManualReference between 0 and 1
      | Tempreature between 0 and 100
      | EmergencyButton = 0 | 1
      | LiquidLevel between 0 and 1 (hmax)
  note: Inputs For Tank2
  note: NAMES
      | --------------------------------------------
      | CT1 = ControlType Tank 1
      | F1 = Fill Tank 1
      | E1 = Empty Tank 1
      | MR1 = Manual Reference Tank1
      | T1 = Temperature Tank 1
      | EB1 = Emergency Button Tank 1
      | LL1 = Liquid Level 1
  note: Inputs For Tank3
  note: Inputs For Tank1
  CT2 : Inport
  F2 : Inport  Port=2
  E2 : Inport  Port=3
  T2 : Inport  Port=4
  EB2 : Inport  Port=5
  CT3 : Inport  Port=6
  F3 : Inport  Port=7
  E3 : Inport  Port=8
  MR3 : Inport  Port=9
  T3 : Inport  Port=10
  EB3 : Inport  Port=11
  Tank2 : Subsystem
  Tank3 : Subsystem
  LL2 : Outport
  LL3 : Outport  Port=2
  wires:
  Tank2/1(LL2) -> LL2/1, Tank3/7(LL2)
  Tank3/1(LL3) -> LL3/1, Tank2/6(LL3)
  EB2/1 -> Tank2/5(EB2)
  MR3/1 -> Tank3/4(MR3)
  CT2/1 -> Tank2/1(CT2)
  F2/1 -> Tank2/2(F2)
  E3/1 -> Tank3/3(E3)
  E2/1 -> Tank2/3(E2)
  T2/1 -> Tank2/4(T2)
  CT3/1 -> Tank3/1(CT3)
  F3/1 -> Tank3/2(F3)
  EB3/1 -> Tank3/6(EB3)
  T3/1 -> Tank3/5(T3)

== system c00010M_harness/M171 ==
  note: VALUES
      | ---------------------------------
      | ControlType = 1 | 2 | 3
      | FillTank = 0 | 1
      | EmptyTank = 0 | 1
      | ManualReference between 0 and 1
      | Tempreature between 0 and 100
      | EmergencyButton = 0 | 1
      | LiquidLevel between 0 and 1 (hmax)
  note: Inputs For Tank2
  note: NAMES
      | --------------------------------------------
      | CT1 = ControlType Tank 1
      | F1 = Fill Tank 1
      | E1 = Empty Tank 1
      | MR1 = Manual Reference Tank1
      | T1 = Temperature Tank 1
      | EB1 = Emergency Button Tank 1
      | LL1 = Liquid Level 1
  note: Inputs For Tank3
  note: Inputs For Tank1
  CT2 : Inport
  F2 : Inport  Port=2
  E2 : Inport  Port=3
  T2 : Inport  Port=4
  EB2 : Inport  Port=5
  CT3 : Inport  Port=6
  F3 : Inport  Port=7
  E3 : Inport  Port=8
  MR3 : Inport  Port=9
  T3 : Inport  Port=10
  EB3 : Inport  Port=11
  Tank2 : Subsystem
  Tank3 : Subsystem
  LL2 : Outport
  LL3 : Outport  Port=2
  wires:
  Tank2/1(LL2) -> LL2/1, Tank3/7(LL2)
  Tank3/1(LL3) -> LL3/1, Tank2/6(LL3)
  EB2/1 -> Tank2/5(EB2)
  MR3/1 -> Tank3/4(MR3)
  CT2/1 -> Tank2/1(CT2)
  F2/1 -> Tank2/2(F2)
  E3/1 -> Tank3/3(E3)
  E2/1 -> Tank2/3(E2)
  T2/1 -> Tank2/4(T2)
  CT3/1 -> Tank3/1(CT3)
  F3/1 -> Tank3/2(F3)
  EB3/1 -> Tank3/6(EB3)
  T3/1 -> Tank3/5(T3)

== system c00010M_harness/M172 ==
  note: VALUES
      | ---------------------------------
      | ControlType = 1 | 2 | 3
      | FillTank = 0 | 1
      | EmptyTank = 0 | 1
      | ManualReference between 0 and 1
      | Tempreature between 0 and 100
      | EmergencyButton = 0 | 1
      | LiquidLevel between 0 and 1 (hmax)
  note: Inputs For Tank2
  note: NAMES
      | --------------------------------------------
      | CT1 = ControlType Tank 1
      | F1 = Fill Tank 1
      | E1 = Empty Tank 1
      | MR1 = Manual Reference Tank1
      | T1 = Temperature Tank 1
      | EB1 = Emergency Button Tank 1
      | LL1 = Liquid Level 1
  note: Inputs For Tank3
  note: Inputs For Tank1
  CT2 : Inport
  F2 : Inport  Port=2
  E2 : Inport  Port=3
  T2 : Inport  Port=4
  EB2 : Inport  Port=5
  CT3 : Inport  Port=6
  F3 : Inport  Port=7
  E3 : Inport  Port=8
  MR3 : Inport  Port=9
  T3 : Inport  Port=10
  EB3 : Inport  Port=11
  Tank2 : Subsystem
  Tank3 : Subsystem
  LL2 : Outport
  LL3 : Outport  Port=2
  wires:
  Tank2/1(LL2) -> LL2/1, Tank3/7(LL2)
  Tank3/1(LL3) -> LL3/1, Tank2/6(LL3)
  EB2/1 -> Tank2/5(EB2)
  MR3/1 -> Tank3/4(MR3)
  CT2/1 -> Tank2/1(CT2)
  F2/1 -> Tank2/2(F2)
  E3/1 -> Tank3/3(E3)
  E2/1 -> Tank2/3(E2)
  T2/1 -> Tank2/4(T2)
  CT3/1 -> Tank3/1(CT3)
  F3/1 -> Tank3/2(F3)
  EB3/1 -> Tank3/6(EB3)
  T3/1 -> Tank3/5(T3)

== system c00010M_harness/M173 ==
  note: VALUES
      | ---------------------------------
      | ControlType = 1 | 2 | 3
      | FillTank = 0 | 1
      | EmptyTank = 0 | 1
      | ManualReference between 0 and 1
      | Tempreature between 0 and 100
      | EmergencyButton = 0 | 1
      | LiquidLevel between 0 and 1 (hmax)
  note: Inputs For Tank2
  note: NAMES
      | --------------------------------------------
      | CT1 = ControlType Tank 1
      | F1 = Fill Tank 1
      | E1 = Empty Tank 1
      | MR1 = Manual Reference Tank1
      | T1 = Temperature Tank 1
      | EB1 = Emergency Button Tank 1
      | LL1 = Liquid Level 1
  note: Inputs For Tank3
  note: Inputs For Tank1
  CT2 : Inport
  F2 : Inport  Port=2
  E2 : Inport  Port=3
  T2 : Inport  Port=4
  EB2 : Inport  Port=5
  CT3 : Inport  Port=6
  F3 : Inport  Port=7
  E3 : Inport  Port=8
  MR3 : Inport  Port=9
  T3 : Inport  Port=10
  EB3 : Inport  Port=11
  Tank2 : Subsystem
  Tank3 : Subsystem
  LL2 : Outport
  LL3 : Outport  Port=2
  wires:
  Tank2/1(LL2) -> LL2/1, Tank3/7(LL2)
  Tank3/1(LL3) -> LL3/1, Tank2/6(LL3)
  EB2/1 -> Tank2/5(EB2)
  MR3/1 -> Tank3/4(MR3)
  CT2/1 -> Tank2/1(CT2)
  F2/1 -> Tank2/2(F2)
  E3/1 -> Tank3/3(E3)
  E2/1 -> Tank2/3(E2)
  T2/1 -> Tank2/4(T2)
  CT3/1 -> Tank3/1(CT3)
  F3/1 -> Tank3/2(F3)
  EB3/1 -> Tank3/6(EB3)
  T3/1 -> Tank3/5(T3)

== system c00010M_harness/M174 ==
  note: VALUES
      | ---------------------------------
      | ControlType = 1 | 2 | 3
      | FillTank = 0 | 1
      | EmptyTank = 0 | 1
      | ManualReference between 0 and 1
      | Tempreature between 0 and 100
      | EmergencyButton = 0 | 1
      | LiquidLevel between 0 and 1 (hmax)
  note: Inputs For Tank2
  note: NAMES
      | --------------------------------------------
      | CT1 = ControlType Tank 1
      | F1 = Fill Tank 1
      | E1 = Empty Tank 1
      | MR1 = Manual Reference Tank1
      | T1 = Temperature Tank 1
      | EB1 = Emergency Button Tank 1
      | LL1 = Liquid Level 1
  note: Inputs For Tank3
  note: Inputs For Tank1
  CT2 : Inport
  F2 : Inport  Port=2
  E2 : Inport  Port=3
  T2 : Inport  Port=4
  EB2 : Inport  Port=5
  CT3 : Inport  Port=6
  F3 : Inport  Port=7
  E3 : Inport  Port=8
  MR3 : Inport  Port=9
  T3 : Inport  Port=10
  EB3 : Inport  Port=11
  Tank2 : Subsystem
  Tank3 : Subsystem
  LL2 : Outport
  LL3 : Outport  Port=2
  wires:
  Tank2/1(LL2) -> LL2/1, Tank3/7(LL2)
  Tank3/1(LL3) -> LL3/1, Tank2/6(LL3)
  EB2/1 -> Tank2/5(EB2)
  MR3/1 -> Tank3/4(MR3)
  CT2/1 -> Tank2/1(CT2)
  F2/1 -> Tank2/2(F2)
  E3/1 -> Tank3/3(E3)
  E2/1 -> Tank2/3(E2)
  T2/1 -> Tank2/4(T2)
  CT3/1 -> Tank3/1(CT3)
  F3/1 -> Tank3/2(F3)
  EB3/1 -> Tank3/6(EB3)
  T3/1 -> Tank3/5(T3)

== system c00010M_harness/M175 ==
  note: VALUES
      | ---------------------------------
      | ControlType = 1 | 2 | 3
      | FillTank = 0 | 1
      | EmptyTank = 0 | 1
      | ManualReference between 0 and 1
      | Tempreature between 0 and 100
      | EmergencyButton = 0 | 1
      | LiquidLevel between 0 and 1 (hmax)
  note: Inputs For Tank2
  note: NAMES
      | --------------------------------------------
      | CT1 = ControlType Tank 1
      | F1 = Fill Tank 1
      | E1 = Empty Tank 1
      | MR1 = Manual Reference Tank1
      | T1 = Temperature Tank 1
      | EB1 = Emergency Button Tank 1
      | LL1 = Liquid Level 1
  note: Inputs For Tank3
  note: Inputs For Tank1
  CT2 : Inport
  F2 : Inport  Port=2
  E2 : Inport  Port=3
  T2 : Inport  Port=4
  EB2 : Inport  Port=5
  CT3 : Inport  Port=6
  F3 : Inport  Port=7
  E3 : Inport  Port=8
  MR3 : Inport  Port=9
  T3 : Inport  Port=10
  EB3 : Inport  Port=11
  Tank2 : Subsystem
  Tank3 : Subsystem
  LL2 : Outport
  LL3 : Outport  Port=2
  wires:
  Tank2/1(LL2) -> LL2/1, Tank3/7(LL2)
  Tank3/1(LL3) -> LL3/1, Tank2/6(LL3)
  EB2/1 -> Tank2/5(EB2)
  MR3/1 -> Tank3/4(MR3)
  CT2/1 -> Tank2/1(CT2)
  F2/1 -> Tank2/2(F2)
  E3/1 -> Tank3/3(E3)
  E2/1 -> Tank2/3(E2)
  T2/1 -> Tank2/4(T2)
  CT3/1 -> Tank3/1(CT3)
  F3/1 -> Tank3/2(F3)
  EB3/1 -> Tank3/6(EB3)
  T3/1 -> Tank3/5(T3)

== system c00010M_harness/M176 ==
  note: VALUES
      | ---------------------------------
      | ControlType = 1 | 2 | 3
      | FillTank = 0 | 1
      | EmptyTank = 0 | 1
      | ManualReference between 0 and 1
      | Tempreature between 0 and 100
      | EmergencyButton = 0 | 1
      | LiquidLevel between 0 and 1 (hmax)
  note: Inputs For Tank2
  note: NAMES
      | --------------------------------------------
      | CT1 = ControlType Tank 1
      | F1 = Fill Tank 1
      | E1 = Empty Tank 1
      | MR1 = Manual Reference Tank1
      | T1 = Temperature Tank 1
      | EB1 = Emergency Button Tank 1
      | LL1 = Liquid Level 1
  note: Inputs For Tank3
  note: Inputs For Tank1
  CT2 : Inport
  F2 : Inport  Port=2
  E2 : Inport  Port=3
  T2 : Inport  Port=4
  EB2 : Inport  Port=5
  CT3 : Inport  Port=6
  F3 : Inport  Port=7
  E3 : Inport  Port=8
  MR3 : Inport  Port=9
  T3 : Inport  Port=10
  EB3 : Inport  Port=11
  Tank2 : Subsystem
  Tank3 : Subsystem
  LL2 : Outport
  LL3 : Outport  Port=2
  wires:
  Tank2/1(LL2) -> LL2/1, Tank3/7(LL2)
  Tank3/1(LL3) -> LL3/1, Tank2/6(LL3)
  EB2/1 -> Tank2/5(EB2)
  MR3/1 -> Tank3/4(MR3)
  CT2/1 -> Tank2/1(CT2)
  F2/1 -> Tank2/2(F2)
  E3/1 -> Tank3/3(E3)
  E2/1 -> Tank2/3(E2)
  T2/1 -> Tank2/4(T2)
  CT3/1 -> Tank3/1(CT3)
  F3/1 -> Tank3/2(F3)
  EB3/1 -> Tank3/6(EB3)
  T3/1 -> Tank3/5(T3)

== system c00010M_harness/M177 ==
  note: VALUES
      | ---------------------------------
      | ControlType = 1 | 2 | 3
      | FillTank = 0 | 1
      | EmptyTank = 0 | 1
      | ManualReference between 0 and 1
      | Tempreature between 0 and 100
      | EmergencyButton = 0 | 1
      | LiquidLevel between 0 and 1 (hmax)
  note: Inputs For Tank2
  note: NAMES
      | --------------------------------------------
      | CT1 = ControlType Tank 1
      | F1 = Fill Tank 1
      | E1 = Empty Tank 1
      | MR1 = Manual Reference Tank1
      | T1 = Temperature Tank 1
      | EB1 = Emergency Button Tank 1
      | LL1 = Liquid Level 1
  note: Inputs For Tank3
  note: Inputs For Tank1
  CT2 : Inport
  F2 : Inport  Port=2
  E2 : Inport  Port=3
  T2 : Inport  Port=4
  EB2 : Inport  Port=5
  CT3 : Inport  Port=6
  F3 : Inport  Port=7
  E3 : Inport  Port=8
  MR3 : Inport  Port=9
  T3 : Inport  Port=10
  EB3 : Inport  Port=11
  Tank2 : Subsystem
  Tank3 : Subsystem
  LL2 : Outport
  LL3 : Outport  Port=2
  wires:
  Tank2/1(LL2) -> LL2/1, Tank3/7(LL2)
  Tank3/1(LL3) -> LL3/1, Tank2/6(LL3)
  EB2/1 -> Tank2/5(EB2)
  MR3/1 -> Tank3/4(MR3)
  CT2/1 -> Tank2/1(CT2)
  F2/1 -> Tank2/2(F2)
  E3/1 -> Tank3/3(E3)
  E2/1 -> Tank2/3(E2)
  T2/1 -> Tank2/4(T2)
  CT3/1 -> Tank3/1(CT3)
  F3/1 -> Tank3/2(F3)
  EB3/1 -> Tank3/6(EB3)
  T3/1 -> Tank3/5(T3)

== system c00010M_harness/M178 ==
  note: VALUES
      | ---------------------------------
      | ControlType = 1 | 2 | 3
      | FillTank = 0 | 1
      | EmptyTank = 0 | 1
      | ManualReference between 0 and 1
      | Tempreature between 0 and 100
      | EmergencyButton = 0 | 1
      | LiquidLevel between 0 and 1 (hmax)
  note: Inputs For Tank2
  note: NAMES
      | --------------------------------------------
      | CT1 = ControlType Tank 1
      | F1 = Fill Tank 1
      | E1 = Empty Tank 1
      | MR1 = Manual Reference Tank1
      | T1 = Temperature Tank 1
      | EB1 = Emergency Button Tank 1
      | LL1 = Liquid Level 1
  note: Inputs For Tank3
  note: Inputs For Tank1
  CT2 : Inport
  F2 : Inport  Port=2
  E2 : Inport  Port=3
  T2 : Inport  Port=4
  EB2 : Inport  Port=5
  CT3 : Inport  Port=6
  F3 : Inport  Port=7
  E3 : Inport  Port=8
  MR3 : Inport  Port=9
  T3 : Inport  Port=10
  EB3 : Inport  Port=11
  Tank2 : Subsystem
  Tank3 : Subsystem
  LL2 : Outport
  LL3 : Outport  Port=2
  wires:
  Tank2/1(LL2) -> LL2/1, Tank3/7(LL2)
  Tank3/1(LL3) -> LL3/1, Tank2/6(LL3)
  EB2/1 -> Tank2/5(EB2)
  MR3/1 -> Tank3/4(MR3)
  CT2/1 -> Tank2/1(CT2)
  F2/1 -> Tank2/2(F2)
  E3/1 -> Tank3/3(E3)
  E2/1 -> Tank2/3(E2)
  T2/1 -> Tank2/4(T2)
  CT3/1 -> Tank3/1(CT3)
  F3/1 -> Tank3/2(F3)
  EB3/1 -> Tank3/6(EB3)
  T3/1 -> Tank3/5(T3)

== system c00010M_harness/M179 ==
  note: VALUES
      | ---------------------------------
      | ControlType = 1 | 2 | 3
      | FillTank = 0 | 1
      | EmptyTank = 0 | 1
      | ManualReference between 0 and 1
      | Tempreature between 0 and 100
      | EmergencyButton = 0 | 1
      | LiquidLevel between 0 and 1 (hmax)
  note: Inputs For Tank2
  note: NAMES
      | --------------------------------------------
      | CT1 = ControlType Tank 1
      | F1 = Fill Tank 1
      | E1 = Empty Tank 1
      | MR1 = Manual Reference Tank1
      | T1 = Temperature Tank 1
      | EB1 = Emergency Button Tank 1
      | LL1 = Liquid Level 1
  note: Inputs For Tank3
  note: Inputs For Tank1
  CT2 : Inport
  F2 : Inport  Port=2
  E2 : Inport  Port=3
  T2 : Inport  Port=4
  EB2 : Inport  Port=5
  CT3 : Inport  Port=6
  F3 : Inport  Port=7
  E3 : Inport  Port=8
  MR3 : Inport  Port=9
  T3 : Inport  Port=10
  EB3 : Inport  Port=11
  Tank2 : Subsystem
  Tank3 : Subsystem
  LL2 : Outport
  LL3 : Outport  Port=2
  wires:
  Tank2/1(LL2) -> LL2/1, Tank3/7(LL2)
  Tank3/1(LL3) -> LL3/1, Tank2/6(LL3)
  EB2/1 -> Tank2/5(EB2)
  MR3/1 -> Tank3/4(MR3)
  CT2/1 -> Tank2/1(CT2)
  F2/1 -> Tank2/2(F2)
  E3/1 -> Tank3/3(E3)
  E2/1 -> Tank2/3(E2)
  T2/1 -> Tank2/4(T2)
  CT3/1 -> Tank3/1(CT3)
  F3/1 -> Tank3/2(F3)
  EB3/1 -> Tank3/6(EB3)
  T3/1 -> Tank3/5(T3)

== system c00010M_harness/M180 ==
  note: VALUES
      | ---------------------------------
      | ControlType = 1 | 2 | 3
      | FillTank = 0 | 1
      | EmptyTank = 0 | 1
      | ManualReference between 0 and 1
      | Tempreature between 0 and 100
      | EmergencyButton = 0 | 1
      | LiquidLevel between 0 and 1 (hmax)
  note: Inputs For Tank2
  note: NAMES
      | --------------------------------------------
      | CT1 = ControlType Tank 1
      | F1 = Fill Tank 1
      | E1 = Empty Tank 1
      | MR1 = Manual Reference Tank1
      | T1 = Temperature Tank 1
      | EB1 = Emergency Button Tank 1
      | LL1 = Liquid Level 1
  note: Inputs For Tank3
  note: Inputs For Tank1
  CT2 : Inport
  F2 : Inport  Port=2
  E2 : Inport  Port=3
  T2 : Inport  Port=4
  EB2 : Inport  Port=5
  CT3 : Inport  Port=6
  F3 : Inport  Port=7
  E3 : Inport  Port=8
  MR3 : Inport  Port=9
  T3 : Inport  Port=10
  EB3 : Inport  Port=11
  Tank2 : Subsystem
  Tank3 : Subsystem
  LL2 : Outport
  LL3 : Outport  Port=2
  wires:
  Tank2/1(LL2) -> LL2/1, Tank3/7(LL2)
  Tank3/1(LL3) -> LL3/1, Tank2/6(LL3)
  EB2/1 -> Tank2/5(EB2)
  MR3/1 -> Tank3/4(MR3)
  CT2/1 -> Tank2/1(CT2)
  F2/1 -> Tank2/2(F2)
  E3/1 -> Tank3/3(E3)
  E2/1 -> Tank2/3(E2)
  T2/1 -> Tank2/4(T2)
  CT3/1 -> Tank3/1(CT3)
  F3/1 -> Tank3/2(F3)
  EB3/1 -> Tank3/6(EB3)
  T3/1 -> Tank3/5(T3)

== system c00010M_harness/M181 ==
  note: VALUES
      | ---------------------------------
      | ControlType = 1 | 2 | 3
      | FillTank = 0 | 1
      | EmptyTank = 0 | 1
      | ManualReference between 0 and 1
      | Tempreature between 0 and 100
      | EmergencyButton = 0 | 1
      | LiquidLevel between 0 and 1 (hmax)
  note: Inputs For Tank2
  note: NAMES
      | --------------------------------------------
      | CT1 = ControlType Tank 1
      | F1 = Fill Tank 1
      | E1 = Empty Tank 1
      | MR1 = Manual Reference Tank1
      | T1 = Temperature Tank 1
      | EB1 = Emergency Button Tank 1
      | LL1 = Liquid Level 1
  note: Inputs For Tank3
  note: Inputs For Tank1
  CT2 : Inport
  F2 : Inport  Port=2
  E2 : Inport  Port=3
  T2 : Inport  Port=4
  EB2 : Inport  Port=5
  CT3 : Inport  Port=6
  F3 : Inport  Port=7
  E3 : Inport  Port=8
  MR3 : Inport  Port=9
  T3 : Inport  Port=10
  EB3 : Inport  Port=11
  Tank2 : Subsystem
  Tank3 : Subsystem
  LL2 : Outport
  LL3 : Outport  Port=2
  wires:
  Tank2/1(LL2) -> LL2/1, Tank3/7(LL2)
  Tank3/1(LL3) -> LL3/1, Tank2/6(LL3)
  EB2/1 -> Tank2/5(EB2)
  MR3/1 -> Tank3/4(MR3)
  CT2/1 -> Tank2/1(CT2)
  F2/1 -> Tank2/2(F2)
  E3/1 -> Tank3/3(E3)
  E2/1 -> Tank2/3(E2)
  T2/1 -> Tank2/4(T2)
  CT3/1 -> Tank3/1(CT3)
  F3/1 -> Tank3/2(F3)
  EB3/1 -> Tank3/6(EB3)
  T3/1 -> Tank3/5(T3)

== system c00010M_harness/M182 ==
  note: VALUES
      | ---------------------------------
      | ControlType = 1 | 2 | 3
      | FillTank = 0 | 1
      | EmptyTank = 0 | 1
      | ManualReference between 0 and 1
      | Tempreature between 0 and 100
      | EmergencyButton = 0 | 1
      | LiquidLevel between 0 and 1 (hmax)
  note: Inputs For Tank2
  note: NAMES
      | --------------------------------------------
      | CT1 = ControlType Tank 1
      | F1 = Fill Tank 1
      | E1 = Empty Tank 1
      | MR1 = Manual Reference Tank1
      | T1 = Temperature Tank 1
      | EB1 = Emergency Button Tank 1
      | LL1 = Liquid Level 1
  note: Inputs For Tank3
  note: Inputs For Tank1
  CT2 : Inport
  F2 : Inport  Port=2
  E2 : Inport  Port=3
  T2 : Inport  Port=4
  EB2 : Inport  Port=5
  CT3 : Inport  Port=6
  F3 : Inport  Port=7
  E3 : Inport  Port=8
  MR3 : Inport  Port=9
  T3 : Inport  Port=10
  EB3 : Inport  Port=11
  Tank2 : Subsystem
  Tank3 : Subsystem
  LL2 : Outport
  LL3 : Outport  Port=2
  wires:
  Tank2/1(LL2) -> LL2/1, Tank3/7(LL2)
  Tank3/1(LL3) -> LL3/1, Tank2/6(LL3)
  EB2/1 -> Tank2/5(EB2)
  MR3/1 -> Tank3/4(MR3)
  CT2/1 -> Tank2/1(CT2)
  F2/1 -> Tank2/2(F2)
  E3/1 -> Tank3/3(E3)
  E2/1 -> Tank2/3(E2)
  T2/1 -> Tank2/4(T2)
  CT3/1 -> Tank3/1(CT3)
  F3/1 -> Tank3/2(F3)
  EB3/1 -> Tank3/6(EB3)
  T3/1 -> Tank3/5(T3)

== system c00010M_harness/M183 ==
  note: VALUES
      | ---------------------------------
      | ControlType = 1 | 2 | 3
      | FillTank = 0 | 1
      | EmptyTank = 0 | 1
      | ManualReference between 0 and 1
      | Tempreature between 0 and 100
      | EmergencyButton = 0 | 1
      | LiquidLevel between 0 and 1 (hmax)
  note: Inputs For Tank2
  note: NAMES
      | --------------------------------------------
      | CT1 = ControlType Tank 1
      | F1 = Fill Tank 1
      | E1 = Empty Tank 1
      | MR1 = Manual Reference Tank1
      | T1 = Temperature Tank 1
      | EB1 = Emergency Button Tank 1
      | LL1 = Liquid Level 1
  note: Inputs For Tank3
  note: Inputs For Tank1
  CT2 : Inport
  F2 : Inport  Port=2
  E2 : Inport  Port=3
  T2 : Inport  Port=4
  EB2 : Inport  Port=5
  CT3 : Inport  Port=6
  F3 : Inport  Port=7
  E3 : Inport  Port=8
  MR3 : Inport  Port=9
  T3 : Inport  Port=10
  EB3 : Inport  Port=11
  Tank2 : Subsystem
  Tank3 : Subsystem
  LL2 : Outport
  LL3 : Outport  Port=2
  wires:
  Tank2/1(LL2) -> LL2/1, Tank3/7(LL2)
  Tank3/1(LL3) -> LL3/1, Tank2/6(LL3)
  EB2/1 -> Tank2/5(EB2)
  MR3/1 -> Tank3/4(MR3)
  CT2/1 -> Tank2/1(CT2)
  F2/1 -> Tank2/2(F2)
  E3/1 -> Tank3/3(E3)
  E2/1 -> Tank2/3(E2)
  T2/1 -> Tank2/4(T2)
  CT3/1 -> Tank3/1(CT3)
  F3/1 -> Tank3/2(F3)
  EB3/1 -> Tank3/6(EB3)
  T3/1 -> Tank3/5(T3)

== system c00010M_harness/M184 ==
  note: VALUES
      | ---------------------------------
      | ControlType = 1 | 2 | 3
      | FillTank = 0 | 1
      | EmptyTank = 0 | 1
      | ManualReference between 0 and 1
      | Tempreature between 0 and 100
      | EmergencyButton = 0 | 1
      | LiquidLevel between 0 and 1 (hmax)
  note: Inputs For Tank2
  note: NAMES
      | --------------------------------------------
      | CT1 = ControlType Tank 1
      | F1 = Fill Tank 1
      | E1 = Empty Tank 1
      | MR1 = Manual Reference Tank1
      | T1 = Temperature Tank 1
      | EB1 = Emergency Button Tank 1
      | LL1 = Liquid Level 1
  note: Inputs For Tank3
  note: Inputs For Tank1
  CT2 : Inport
  F2 : Inport  Port=2
  E2 : Inport  Port=3
  T2 : Inport  Port=4
  EB2 : Inport  Port=5
  CT3 : Inport  Port=6
  F3 : Inport  Port=7
  E3 : Inport  Port=8
  MR3 : Inport  Port=9
  T3 : Inport  Port=10
  EB3 : Inport  Port=11
  Tank2 : Subsystem
  Tank3 : Subsystem
  LL2 : Outport
  LL3 : Outport  Port=2
  wires:
  Tank2/1(LL2) -> LL2/1, Tank3/7(LL2)
  Tank3/1(LL3) -> LL3/1, Tank2/6(LL3)
  EB2/1 -> Tank2/5(EB2)
  MR3/1 -> Tank3/4(MR3)
  CT2/1 -> Tank2/1(CT2)
  F2/1 -> Tank2/2(F2)
  E3/1 -> Tank3/3(E3)
  E2/1 -> Tank2/3(E2)
  T2/1 -> Tank2/4(T2)
  CT3/1 -> Tank3/1(CT3)
  F3/1 -> Tank3/2(F3)
  EB3/1 -> Tank3/6(EB3)
  T3/1 -> Tank3/5(T3)

== system c00010M_harness/M185 ==
  note: VALUES
      | ---------------------------------
      | ControlType = 1 | 2 | 3
      | FillTank = 0 | 1
      | EmptyTank = 0 | 1
      | ManualReference between 0 and 1
      | Tempreature between 0 and 100
      | EmergencyButton = 0 | 1
      | LiquidLevel between 0 and 1 (hmax)
  note: Inputs For Tank2
  note: NAMES
      | --------------------------------------------
      | CT1 = ControlType Tank 1
      | F1 = Fill Tank 1
      | E1 = Empty Tank 1
      | MR1 = Manual Reference Tank1
      | T1 = Temperature Tank 1
      | EB1 = Emergency Button Tank 1
      | LL1 = Liquid Level 1
  note: Inputs For Tank3
  note: Inputs For Tank1
  CT2 : Inport
  F2 : Inport  Port=2
  E2 : Inport  Port=3
  T2 : Inport  Port=4
  EB2 : Inport  Port=5
  CT3 : Inport  Port=6
  F3 : Inport  Port=7
  E3 : Inport  Port=8
  MR3 : Inport  Port=9
  T3 : Inport  Port=10
  EB3 : Inport  Port=11
  Tank2 : Subsystem
  Tank3 : Subsystem
  LL2 : Outport
  LL3 : Outport  Port=2
  wires:
  Tank2/1(LL2) -> LL2/1, Tank3/7(LL2)
  Tank3/1(LL3) -> LL3/1, Tank2/6(LL3)
  EB2/1 -> Tank2/5(EB2)
  MR3/1 -> Tank3/4(MR3)
  CT2/1 -> Tank2/1(CT2)
  F2/1 -> Tank2/2(F2)
  E3/1 -> Tank3/3(E3)
  E2/1 -> Tank2/3(E2)
  T2/1 -> Tank2/4(T2)
  CT3/1 -> Tank3/1(CT3)
  F3/1 -> Tank3/2(F3)
  EB3/1 -> Tank3/6(EB3)
  T3/1 -> Tank3/5(T3)
